simulink model "IEEE34BARRAS"  (R2018a)
settings: Solver=ode4  StartTime=0.0  StopTime=48*T  FixedStep=Ts  RelTol=1e-3  EnableMultiTasking=on
InitFcn:
  | close
  | clc
  | clear
  | n=2^8;
  | f=60;
  | T=1/f;
  | Ts=1/(f*n);
  | NT=18;
  | set_param('IEEE34BARRAS/EMISOR-RECEPTOR/TCP_IP_RX1/ESCRITURA', 'Value','[0,0,0,0,0,0,0,0,0,0,0,0,0,0,0,0,0,0,0,0,0,0,0,0,0,0,0,0,0,0,0,0,0,0,0,0,0,0,0,0,0]')
  | set_param('IEEE34BARRAS/EMISOR-RECEPTOR/TCP_IP_RX1/RETARDO', 'Value','0')
  | run script_client_1_inicio1.m
undefined symbols (not defined in the file or in its folder): D1, Delta, DiscIntNeverNeededParam, Ip1
libraries: powerlib x313, simulink x15, libreria_medidores1T x3, libreria_comunicaciones_cliente1T x2
(part 1 of 5)
settings Model: Creator=Juan Antonio Ocampo  LastModifiedBy=ana-n
settings DataIOCC: LimitDataPoints=on
settings OptimizationCC: LifeSpan=inf
settings DebuggingCC: AllowSymbolicDim=off  SFUnexpectedBacktrackingDiag=warning  SFNoUnconditionalDefaultTransitionDiag=warning  SFExecutionAtInitializationDiag=none
settings ModelReferenceCC: PropagateSignalLabelsOutOfModel=off
settings CodeAppCC: StateflowObjectComments=on
settings GRTTargetCC: TargetLangStandard=C89/C90 (ANSI)
settings ConfigComp: CovMetricSettings=dw  CovHtmlReporting=on  CovSaveCumulativeToWorkspaceVar=on  CovSaveSingleToWorkspaceVar=on  CovExternalEMLEnable=off
settings SimscapeCC: SimscapeNormalizeSystem=off

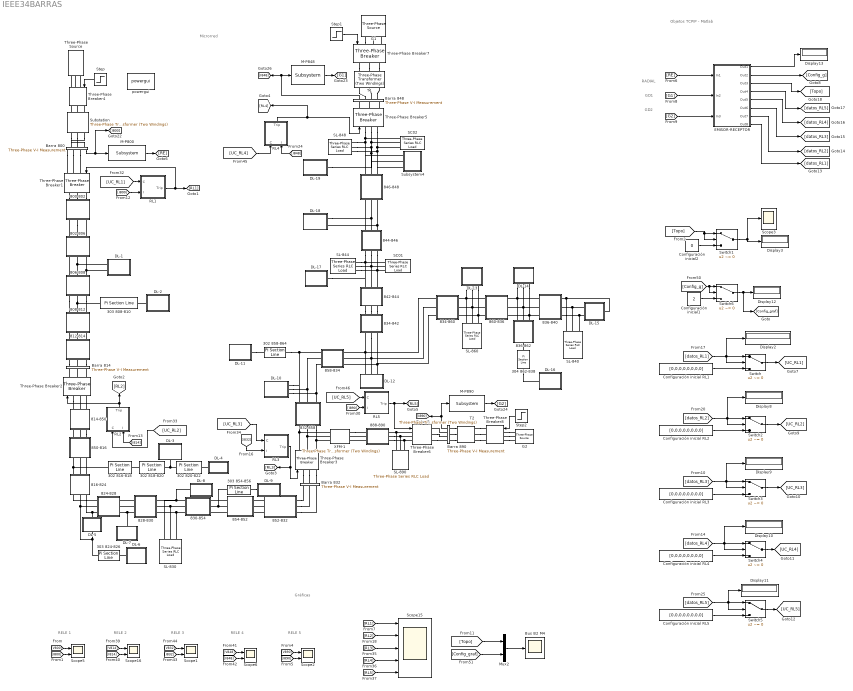
== system IEEE34BARRAS ==
  note: RADIAL
  note: RELE 1
  note: RELE 2
  note: RELE 3
  note: RELE 5
  note: RELE 4
  note: Gráficas
  note: Microrred
  note: Objetos TCPIP - Matlab
  note: GD1
  note: GD2
  " G1" : powerlib/Electrical Sources/Three-Phase Source  InternalConnection=Yg  VoltagePhases=on  Voltage=10e3/sqrt(2)  PhaseAngle=0  Voltage_phases=[480 480 480]/sqrt(3)  PhaseAngles_phases=[0 -120 +120]  Frequency=60  NonIdealSource=on  SpecifyImpedance=on  Resistance=0.8929  Inductance=16.58e-3  ShortCircuitLevel=100e6  BaseVoltage=480  XRratio=1  BusType=swing  Pref=2.324  Qref=-0.169  Prefabc=1000e6*[1 1 1]  Qrefabc=[0, 0, 0]  Qmin=0  Qmax=0
  " G2" : powerlib/Electrical Sources/Three-Phase Source  InternalConnection=Yg  VoltagePhases=on  Voltage=10e3/sqrt(2)  PhaseAngle=0  Voltage_phases=[480 480 480]  PhaseAngles_phases=[0 -120 +120]  Frequency=60  NonIdealSource=on  SpecifyImpedance=on  Resistance=0.8929  Inductance=16.58e-3  ShortCircuitLevel=100e6  BaseVoltage=480  XRratio=1  BusType=swing  Pref=2.324  Qref=-0.169  Prefabc=1000e6*[1 1 1]  Qrefabc=[0, 0, 0]  Qmin=0  Qmax=0
  302 816-818 : powerlib/Elements/Pi Section Line  LConnTagsString=__new0  RConnTagsString=__new0  Frequency=60  Resistance=1.7396  Inductance=0.0024  Capacitance=0.0070*1e-6  Length=0.5212  PiSections=1  Measurements=None
      settings: AttributesFormatString=\n  SourceProductName=Simscape Power Systems  SourceProductBaseCode=PS
  302 818-820 : powerlib/Elements/Pi Section Line  LConnTagsString=__new0  RConnTagsString=__new0  Frequency=60  Resistance=1.7396  Inductance=0.0024  Capacitance=0.0070*1e-6  Length=14.6761  PiSections=1  Measurements=None
      settings: AttributesFormatString=\n  SourceProductName=Simscape Power Systems  SourceProductBaseCode=PS
  302 820-822 : powerlib/Elements/Pi Section Line  LConnTagsString=__new0  RConnTagsString=__new0  Frequency=60  Resistance=1.7396  Inductance=0.0024  Capacitance=0.0070*1e-6  Length=4.1880  PiSections=1  Measurements=None
      settings: AttributesFormatString=\n  SourceProductName=Simscape Power Systems  SourceProductBaseCode=PS
  302 858-864 : powerlib/Elements/Pi Section Line  LConnTagsString=__new0  RConnTagsString=__new0  Frequency=60  Resistance=1.7396  Inductance=0.0024  Capacitance=0.0070*1e-6  Length=0.4938  PiSections=1  Measurements=None
      settings: AttributesFormatString=\n  SourceProductName=Simscape Power Systems  SourceProductBaseCode=PS
  303 808-810 : powerlib/Elements/Pi Section Line  LConnTagsString=__new0  RConnTagsString=__new0  Frequency=60  Resistance=1.7396  Inductance=0.0024  Capacitance=0.0070*1e-6  Length=1.769059  PiSections=1  Measurements=None
      settings: AttributesFormatString=\n  SourceProductName=Simscape Power Systems  SourceProductBaseCode=PS
  303 824-826 : powerlib/Elements/Pi Section Line  LConnTagsString=__new0  RConnTagsString=__new0  Frequency=60  Resistance=1.7396  Inductance=0.0024  Capacitance=0.0070*1e-6  Length=1.769059  PiSections=1  Measurements=None
      settings: AttributesFormatString=\n  SourceProductName=Simscape Power Systems  SourceProductBaseCode=PS
  303 854-856 : powerlib/Elements/Pi Section Line  LConnTagsString=__new0  RConnTagsString=__new0  Frequency=60  Resistance=1.7396  Inductance=0.0024  Capacitance=0.0070*1e-6  Length=7.111  PiSections=1  Measurements=None
      settings: AttributesFormatString=\n  SourceProductName=Simscape Power Systems  SourceProductBaseCode=PS
  304 862-838 : powerlib/Elements/Pi Section Line  LConnTagsString=__new0  RConnTagsString=__new0  Frequency=60  Resistance=1.1941  Inductance=0.0023  Capacitance=0.0072*1e-6  Length=1.769059  PiSections=1  Measurements=None
      settings: AttributesFormatString=\n  SourceProductName=Simscape Power Systems  SourceProductBaseCode=PS
  800-802 : Subsystem  mask{Ft=0.4886364, R=[0.8307,0.8226,0.8361], L=[0.0022,0.0022,0.0022], C=[0.0088,0.0084,0.0081].*1e-6}
      mask prompts: Ft "Distancia"; R "Resistencia p"; L "Inductancia p"; C "Capacitancia p"
      mask Display:
      | plot(0,0,100,100,[20,20,80,80,90,80,80,20,20,10],[50,40,40,50,50,50,61,61,50,50],[56,39],[55,55],[44,44],[44,55],[53,50,50],[44,48,55])
      | text(50,30,'300', 'horizontalAlignment', 'center');
      | port_label('RConn', 1, 'a')
      | port_label('RConn', 2, 'b')
      | port_label('RConn', 3, 'c')
      | port_label('LConn', 1, 'A')
      | port_label('LConn', 2, 'B')
      | port_label('LConn', 3, 'C')
  802-806 : Subsystem  mask{Ft=0.3276515, R=[0.8307,0.8226,0.8361], L=[0.0022,0.0022,0.0022], C=[0.0088,0.0084,0.0081].*1e-6}
      mask prompts: Ft "Distancia"; R "Resistencia p"; L "Inductancia p"; C "Capacitancia p"
      mask Display:
      | plot(0,0,100,100,[20,20,80,80,90,80,80,20,20,10],[50,40,40,50,50,50,61,61,50,50],[56,39],[55,55],[44,44],[44,55],[53,50,50],[44,48,55])
      | text(50,30,'300', 'horizontalAlignment', 'center');
      | port_label('RConn', 1, 'a')
      | port_label('RConn', 2, 'b')
      | port_label('RConn', 3, 'c')
      | port_label('LConn', 1, 'A')
      | port_label('LConn', 2, 'B')
      | port_label('LConn', 3, 'C')
  806-808 : Subsystem  mask{Ft=6.1041667, R=[0.8307,0.8226,0.8361], L=[0.0022,0.0022,0.0022], C=[0.0088,0.0084,0.0081].*1e-6}
      mask prompts: Ft "Distancia"; R "Resistencia p"; L "Inductancia p"; C "Capacitancia p"
      mask Display:
      | plot(0,0,100,100,[20,20,80,80,90,80,80,20,20,10],[50,40,40,50,50,50,61,61,50,50],[56,39],[55,55],[44,44],[44,55],[53,50,50],[44,48,55])
      | text(50,30,'300', 'horizontalAlignment', 'center');
      | port_label('RConn', 1, 'a')
      | port_label('RConn', 2, 'b')
      | port_label('RConn', 3, 'c')
      | port_label('LConn', 1, 'A')
      | port_label('LConn', 2, 'B')
      | port_label('LConn', 3, 'C')
  808-812 : Subsystem  mask{Ft=7.1022727, R=[0.8307,0.8226,0.8361], L=[0.0022,0.0022,0.0022], C=[0.0088,0.0084,0.0081].*1e-6}
      mask prompts: Ft "Distancia"; R "Resistencia p"; L "Inductancia p"; C "Capacitancia p"
      mask Display:
      | plot(0,0,100,100,[20,20,80,80,90,80,80,20,20,10],[50,40,40,50,50,50,61,61,50,50],[56,39],[55,55],[44,44],[44,55],[53,50,50],[44,48,55])
      | text(50,30,'300', 'horizontalAlignment', 'center');
      | port_label('RConn', 1, 'a')
      | port_label('RConn', 2, 'b')
      | port_label('RConn', 3, 'c')
      | port_label('LConn', 1, 'A')
      | port_label('LConn', 2, 'B')
      | port_label('LConn', 3, 'C')
  812-814 : Subsystem  mask{Ft=5.6306818, R=[0.8307,0.8226,0.8361], L=[0.0022,0.0022,0.0022], C=[0.0088,0.0084,0.0081].*1e-6}
      mask prompts: Ft "Distancia"; R "Resistencia p"; L "Inductancia p"; C "Capacitancia p"
      mask Display:
      | plot(0,0,100,100,[20,20,80,80,90,80,80,20,20,10],[50,40,40,50,50,50,61,61,50,50],[56,39],[55,55],[44,44],[44,55],[53,50,50],[44,48,55])
      | text(50,30,'300', 'horizontalAlignment', 'center');
      | port_label('RConn', 1, 'a')
      | port_label('RConn', 2, 'b')
      | port_label('RConn', 3, 'c')
      | port_label('LConn', 1, 'A')
      | port_label('LConn', 2, 'B')
      | port_label('LConn', 3, 'C')
  814-850 : Subsystem  mask{Ft=0.00189394, R=[1.1993,1.1904,1.1943], L=[0.0023,0.0024,0.0023], C=[0.0084,0.0081,0.0078].*1e-6}
      mask prompts: Ft "Distancia"; R "Resistencia p"; L "Inductancia p"; C "Capacitancia p"
      mask Display:
      | plot(0,0,100,100,[20,20,80,80,90,80,80,20,20,10],[50,40,40,50,50,50,61,61,50,50],[56,39],[55,55],[44,44],[44,55],[53,50,50],[44,48,55])
      | text(50,30,'301', 'horizontalAlignment', 'center');
      | port_label('RConn', 1, 'a')
      | port_label('RConn', 2, 'b')
      | port_label('RConn', 3, 'c')
      | port_label('LConn', 1, 'A')
      | port_label('LConn', 2, 'B')
      | port_label('LConn', 3, 'C')
  816-824 : Subsystem  mask{Ft=1.9337121, R=[1.1993,1.1904,1.1943], L=[0.0023,0.0024,0.0023], C=[0.0084,0.0081,0.0078].*1e-6}
      mask prompts: Ft "Distancia"; R "Resistencia p"; L "Inductancia p"; C "Capacitancia p"
      mask Display:
      | plot(0,0,100,100,[20,20,80,80,90,80,80,20,20,10],[50,40,40,50,50,50,61,61,50,50],[56,39],[55,55],[44,44],[44,55],[53,50,50],[44,48,55])
      | text(50,30,'301', 'horizontalAlignment', 'center');
      | port_label('RConn', 1, 'a')
      | port_label('RConn', 2, 'b')
      | port_label('RConn', 3, 'c')
      | port_label('LConn', 1, 'A')
      | port_label('LConn', 2, 'B')
      | port_label('LConn', 3, 'C')
  824-828 : Subsystem  mask{Ft=0.159091, R=[1.1993,1.1904,1.1943], L=[0.0023,0.0024,0.0023], C=[0.0084,0.0081,0.0078].*1e-6}
      mask prompts: Ft "Distancia"; R "Resistencia p"; L "Inductancia p"; C "Capacitancia p"
      mask Display:
      | plot(0,0,100,100,[20,20,80,80,90,80,80,20,20,10],[50,40,40,50,50,50,61,61,50,50],[56,39],[55,55],[44,44],[44,55],[53,50,50],[44,48,55])
      | text(50,30,'301', 'horizontalAlignment', 'center');
      | port_label('RConn', 1, 'a')
      | port_label('RConn', 2, 'b')
      | port_label('RConn', 3, 'c')
      | port_label('LConn', 1, 'A')
      | port_label('LConn', 2, 'B')
      | port_label('LConn', 3, 'C')
  828-830 : Subsystem  mask{Ft=3.8712121, R=[1.1081,1.1081,1.1081,1.1082], L=[0.0026858,0.0026858,0.0026858,0.0026853], C=[3.5034e-09,3.0270e-09,3.8602e-09,3.7929e-09]}
      mask prompts: Ft "Distancia"; R "Resistencia p"; L "Inductancia p"; C "Capacitancia p"
      mask Display:
      | plot(0,0,100,100,[20,20,80,80,90,80,80,20,20,10],[50,40,40,50,50,50,61,61,50,50],[56,39],[55,55],[44,44],[44,55],[53,50,50],[44,48,55])
      | text(50,30,'301', 'horizontalAlignment', 'center');
      | port_label('RConn', 1, 'a')
      | port_label('RConn', 2, 'b')
      | port_label('RConn', 3, 'c')
      | port_label('LConn', 1, 'A')
      | port_label('LConn', 2, 'B')
      | port_label('LConn', 3, 'C')
  830-854 : Subsystem  mask{Ft=0.0984848, R=[1.1993,1.1904,1.1943], L=[0.0023,0.0024,0.0023], C=[0.0084,0.0081,0.0078].*1e-6}
      mask prompts: Ft "Distancia"; R "Resistencia p"; L "Inductancia p"; C "Capacitancia p"
      mask Display:
      | plot(0,0,100,100,[20,20,80,80,90,80,80,20,20,10],[50,40,40,50,50,50,61,61,50,50],[56,39],[55,55],[44,44],[44,55],[53,50,50],[44,48,55])
      | text(50,30,'301', 'horizontalAlignment', 'center');
      | port_label('RConn', 1, 'a')
      | port_label('RConn', 2, 'b')
      | port_label('RConn', 3, 'c')
      | port_label('LConn', 1, 'A')
      | port_label('LConn', 2, 'B')
      | port_label('LConn', 3, 'C')
  832-858 : Subsystem  mask{Ft=0.9280303, R=[1.1993,1.1904,1.1943], L=[0.0023,0.0024,0.0023], C=[0.0084,0.0081,0.0078].*1e-6}
      mask prompts: Ft "Distancia"; R "Resistencia p"; L "Inductancia p"; C "Capacitancia p"
      mask Display:
      | plot(0,0,100,100,[20,20,80,80,90,80,80,20,20,10],[50,40,40,50,50,50,61,61,50,50],[56,39],[55,55],[44,44],[44,55],[53,50,50],[44,48,55])
      | text(50,30,'301', 'horizontalAlignment', 'center');
      | port_label('RConn', 1, 'a')
      | port_label('RConn', 2, 'b')
      | port_label('RConn', 3, 'c')
      | port_label('LConn', 1, 'A')
      | port_label('LConn', 2, 'B')
      | port_label('LConn', 3, 'C')
  834-842 : Subsystem  mask{Ft=0.0530303, R=[1.1993,1.1904,1.1943], L=[0.0023,0.0024,0.0023], C=[0.0084,0.0081,0.0078].*1e-6}
      mask prompts: Ft "Distancia"; R "Resistencia p"; L "Inductancia p"; C "Capacitancia p"
      mask Display:
      | plot(0,0,100,100,[20,20,80,80,90,80,80,20,20,10],[50,40,40,50,50,50,61,61,50,50],[56,39],[55,55],[44,44],[44,55],[53,50,50],[44,48,55])
      | text(50,30,'301', 'horizontalAlignment', 'center');
      | port_label('RConn', 1, 'a')
      | port_label('RConn', 2, 'b')
      | port_label('RConn', 3, 'c')
      | port_label('LConn', 1, 'A')
      | port_label('LConn', 2, 'B')
      | port_label('LConn', 3, 'C')
  834-860 : Subsystem  mask{Ft=0.3825758, R=[1.1993,1.1904,1.1943], L=[0.0023,0.0024,0.0023], C=[0.0084,0.0081,0.0078].*1e-6}
      mask prompts: Ft "Distancia"; R "Resistencia p"; L "Inductancia p"; C "Capacitancia p"
      mask Display:
      | plot(0,0,100,100,[20,20,80,80,90,80,80,20,20,10],[50,40,40,50,50,50,61,61,50,50],[56,39],[55,55],[44,44],[44,55],[53,50,50],[44,48,55])
      | text(50,30,'301', 'horizontalAlignment', 'center');
      | port_label('RConn', 1, 'a')
      | port_label('RConn', 2, 'b')
      | port_label('RConn', 3, 'c')
      | port_label('LConn', 1, 'A')
      | port_label('LConn', 2, 'B')
      | port_label('LConn', 3, 'C')
  836-840 : Subsystem  mask{Ft=0.162879, R=[1.1993,1.1904,1.1943], L=[0.0023,0.0024,0.0023], C=[0.0084,0.0081,0.0078].*1e-6}
      mask prompts: Ft "Distancia"; R "Resistencia p"; L "Inductancia p"; C "Capacitancia p"
      mask Display:
      | plot(0,0,100,100,[20,20,80,80,90,80,80,20,20,10],[50,40,40,50,50,50,61,61,50,50],[56,39],[55,55],[44,44],[44,55],[53,50,50],[44,48,55])
      | text(50,30,'301', 'horizontalAlignment', 'center');
      | port_label('RConn', 1, 'a')
      | port_label('RConn', 2, 'b')
      | port_label('RConn', 3, 'c')
      | port_label('LConn', 1, 'A')
      | port_label('LConn', 2, 'B')
      | port_label('LConn', 3, 'C')
  836-862 : Subsystem  mask{Ft=0.0530303, R=[1.1993,1.1904,1.1943], L=[0.0023,0.0024,0.0023], C=[0.0084,0.0081,0.0078].*1e-6}
      mask prompts: Ft "Distancia"; R "Resistencia p"; L "Inductancia p"; C "Capacitancia p"
      mask Display:
      | plot(0,0,100,100,[20,20,80,80,90,80,80,20,20,10],[50,40,40,50,50,50,61,61,50,50],[56,39],[55,55],[44,44],[44,55],[53,50,50],[44,48,55])
      | text(50,30,'301', 'horizontalAlignment', 'center');
      | port_label('RConn', 1, 'a')
      | port_label('RConn', 2, 'b')
      | port_label('RConn', 3, 'c')
      | port_label('LConn', 1, 'A')
      | port_label('LConn', 2, 'B')
      | port_label('LConn', 3, 'C')
  842-844 : Subsystem  mask{Ft=0.2556818, R=[1.1993,1.1904,1.1943], L=[0.0023,0.0024,0.0023], C=[0.0084,0.0081,0.0078].*1e-6}
      mask prompts: Ft "Distancia"; R "Resistencia p"; L "Inductancia p"; C "Capacitancia p"
      mask Display:
      | plot(0,0,100,100,[20,20,80,80,90,80,80,20,20,10],[50,40,40,50,50,50,61,61,50,50],[56,39],[55,55],[44,44],[44,55],[53,50,50],[44,48,55])
      | text(50,30,'301', 'horizontalAlignment', 'center');
      | port_label('RConn', 1, 'a')
      | port_label('RConn', 2, 'b')
      | port_label('RConn', 3, 'c')
      | port_label('LConn', 1, 'A')
      | port_label('LConn', 2, 'B')
      | port_label('LConn', 3, 'C')
  844-846 : Subsystem  mask{Ft=0.6893939, R=[1.1993,1.1904,1.1943], L=[0.0023,0.0024,0.0023], C=[0.0084,0.0081,0.0078].*1e-6}
      mask prompts: Ft "Distancia"; R "Resistencia p"; L "Inductancia p"; C "Capacitancia p"
      mask Display:
      | plot(0,0,100,100,[20,20,80,80,90,80,80,20,20,10],[50,40,40,50,50,50,61,61,50,50],[56,39],[55,55],[44,44],[44,55],[53,50,50],[44,48,55])
      | text(50,30,'301', 'horizontalAlignment', 'center');
      | port_label('RConn', 1, 'a')
      | port_label('RConn', 2, 'b')
      | port_label('RConn', 3, 'c')
      | port_label('LConn', 1, 'A')
      | port_label('LConn', 2, 'B')
      | port_label('LConn', 3, 'C')
  846-848 : Subsystem  mask{Ft=0.100379, R=[1.1993,1.1904,1.1943], L=[0.0023,0.0024,0.0023], C=[0.0084,0.0081,0.0078].*1e-6}
      mask prompts: Ft "Distancia"; R "Resistencia p"; L "Inductancia p"; C "Capacitancia p"
      mask Display:
      | plot(0,0,100,100,[20,20,80,80,90,80,80,20,20,10],[50,40,40,50,50,50,61,61,50,50],[56,39],[55,55],[44,44],[44,55],[53,50,50],[44,48,55])
      | text(50,30,'301', 'horizontalAlignment', 'center');
      | port_label('RConn', 1, 'a')
      | port_label('RConn', 2, 'b')
      | port_label('RConn', 3, 'c')
      | port_label('LConn', 1, 'A')
      | port_label('LConn', 2, 'B')
      | port_label('LConn', 3, 'C')
  850-816 : Subsystem  mask{Ft=0.0587121, R=[1.1993,1.1904,1.1943], L=[0.0023,0.0024,0.0023], C=[0.0084,0.0081,0.0078].*1e-6}
      mask prompts: Ft "Distancia"; R "Resistencia p"; L "Inductancia p"; C "Capacitancia p"
      mask Display:
      | plot(0,0,100,100,[20,20,80,80,90,80,80,20,20,10],[50,40,40,50,50,50,61,61,50,50],[56,39],[55,55],[44,44],[44,55],[53,50,50],[44,48,55])
      | text(50,30,'301', 'horizontalAlignment', 'center');
      | port_label('RConn', 1, 'a')
      | port_label('RConn', 2, 'b')
      | port_label('RConn', 3, 'c')
      | port_label('LConn', 1, 'A')
      | port_label('LConn', 2, 'B')
      | port_label('LConn', 3, 'C')
  852-832 : Subsystem  mask{Ft=0.00189394, R=[1.1993,1.1904,1.1943], L=[0.0023,0.0024,0.0023], C=[0.0084,0.0081,0.0078].*1e-6}
      mask prompts: Ft "Distancia"; R "Resistencia p"; L "Inductancia p"; C "Capacitancia p"
      mask Display:
      | plot(0,0,100,100,[20,20,80,80,90,80,80,20,20,10],[50,40,40,50,50,50,61,61,50,50],[56,39],[55,55],[44,44],[44,55],[53,50,50],[44,48,55])
      | text(50,30,'301', 'horizontalAlignment', 'center');
      | port_label('RConn', 1, 'a')
      | port_label('RConn', 2, 'b')
      | port_label('RConn', 3, 'c')
      | port_label('LConn', 1, 'A')
      | port_label('LConn', 2, 'B')
      | port_label('LConn', 3, 'C')
  854-852 : Subsystem  mask{Ft=6.9753788, R=[1.1993,1.1904,1.1943], L=[0.0023,0.0024,0.0023], C=[0.0084,0.0081,0.0078].*1e-6}
      mask prompts: Ft "Distancia"; R "Resistencia p"; L "Inductancia p"; C "Capacitancia p"
      mask Display:
      | plot(0,0,100,100,[20,20,80,80,90,80,80,20,20,10],[50,40,40,50,50,50,61,61,50,50],[56,39],[55,55],[44,44],[44,55],[53,50,50],[44,48,55])
      | text(50,30,'301', 'horizontalAlignment', 'center');
      | port_label('RConn', 1, 'a')
      | port_label('RConn', 2, 'b')
      | port_label('RConn', 3, 'c')
      | port_label('LConn', 1, 'A')
      | port_label('LConn', 2, 'B')
      | port_label('LConn', 3, 'C')
  858-834 : Subsystem  mask{Ft=1.104167, R=[1.1993,1.1904,1.1943], L=[0.0023,0.0024,0.0023], C=[0.0084,0.0081,0.0078].*1e-6}
      mask prompts: Ft "Distancia"; R "Resistencia p"; L "Inductancia p"; C "Capacitancia p"
      mask Display:
      | plot(0,0,100,100,[20,20,80,80,90,80,80,20,20,10],[50,40,40,50,50,50,61,61,50,50],[56,39],[55,55],[44,44],[44,55],[53,50,50],[44,48,55])
      | text(50,30,'301', 'horizontalAlignment', 'center');
      | port_label('RConn', 1, 'a')
      | port_label('RConn', 2, 'b')
      | port_label('RConn', 3, 'c')
      | port_label('LConn', 1, 'A')
      | port_label('LConn', 2, 'B')
      | port_label('LConn', 3, 'C')
  860-836 : Subsystem  mask{Ft=0.5075758, R=[1.1993,1.1904,1.1943], L=[0.0023,0.0024,0.0023], C=[0.0084,0.0081,0.0078].*1e-6}
      mask prompts: Ft "Distancia"; R "Resistencia p"; L "Inductancia p"; C "Capacitancia p"
      mask Display:
      | plot(0,0,100,100,[20,20,80,80,90,80,80,20,20,10],[50,40,40,50,50,50,61,61,50,50],[56,39],[55,55],[44,44],[44,55],[53,50,50],[44,48,55])
      | text(50,30,'301', 'horizontalAlignment', 'center');
      | port_label('RConn', 1, 'a')
      | port_label('RConn', 2, 'b')
      | port_label('RConn', 3, 'c')
      | port_label('LConn', 1, 'A')
      | port_label('LConn', 2, 'B')
      | port_label('LConn', 3, 'C')
  888-890 : Subsystem  mask{Ft=2, R=[0.8307,0.8226,0.8361], L=[0.0022,0.0022,0.0022], C=[0.0088,0.0084,0.0081].*1e-6}
      mask prompts: Ft "Distancia"; R "Resistencia p"; L "Inductancia p"; C "Capacitancia p"
      mask Display:
      | plot(0,0,100,100,[20,20,80,80,90,80,80,20,20,10],[50,40,40,50,50,50,61,61,50,50],[56,39],[55,55],[44,44],[44,55],[53,50,50],[44,48,55])
      | text(50,30,'300', 'horizontalAlignment', 'center');
      | port_label('RConn', 1, 'a')
      | port_label('RConn', 2, 'b')
      | port_label('RConn', 3, 'c')
      | port_label('LConn', 1, 'A')
      | port_label('LConn', 2, 'B')
      | port_label('LConn', 3, 'C')
  Barra 800 : powerlib/Measurements/Three-Phase V-I Measurement  VoltageMeasurement=phase-to-phase  SetLabelV=on  LabelV=V800  Vpu=off  VpuLL=off  CurrentMeasurement=yes  SetLabelI=off  LabelI=I800  Ipu=off  Pbase=100e6  Vbase=500e3  OutputType=Complex  PhasorSimulation=off  PSBequivalent=0
  Barra 814 : powerlib/Measurements/Three-Phase V-I Measurement  VoltageMeasurement=phase-to-phase  SetLabelV=on  LabelV=V814  Vpu=off  VpuLL=off  CurrentMeasurement=yes  SetLabelI=on  LabelI=I814  Ipu=off  Pbase=100e6  Vbase=500e3  OutputType=Complex  PhasorSimulation=off  PSBequivalent=0
  Barra 832 : powerlib/Measurements/Three-Phase V-I Measurement  VoltageMeasurement=phase-to-phase  SetLabelV=on  LabelV=V832  Vpu=off  VpuLL=off  CurrentMeasurement=yes  SetLabelI=on  LabelI=I832  Ipu=off  Pbase=100e6  Vbase=500e3  OutputType=Complex  PhasorSimulation=off  PSBequivalent=0
  Barra 848 : powerlib/Measurements/Three-Phase V-I Measurement  VoltageMeasurement=phase-to-phase  SetLabelV=on  LabelV=V848  Vpu=off  VpuLL=off  CurrentMeasurement=yes  SetLabelI=off  LabelI=I848  Ipu=off  Pbase=100e6  Vbase=500e3  OutputType=Complex  PhasorSimulation=off  PSBequivalent=0
  Barra 890 : powerlib/Measurements/Three-Phase V-I Measurement  VoltageMeasurement=phase-to-phase  SetLabelV=on  LabelV=V890  Vpu=off  VpuLL=off  CurrentMeasurement=yes  SetLabelI=off  LabelI=I890  Ipu=off  Pbase=100e6  Vbase=500e3  OutputType=Complex  PhasorSimulation=off  PSBequivalent=0
  Bus B2 M4 : Scope
  Configuración inicial RL{1..5} (5 alike) : Constant  Value=[0,0,0,0,0,0,0,0]
  Configuración inicial1 : Constant  Value=2
  Configuración inicial2 : Constant  Value=0
  DL-1 : Subsystem
      mask Display: disp('802-806')
  DL-10 : Subsystem
      mask Display: disp('832-858')
  DL-11 : Subsystem
      mask Display: disp('858-864')
  DL-12 : Subsystem
      mask Display: disp('858-834')
  DL-13 : Subsystem
      mask Display: disp('834-860')
  DL-14 : Subsystem
      mask Display: disp('860-836')
  DL-15 : Subsystem
      mask Display: disp('836-840')
  DL-16 : Subsystem
      mask Display: disp('862-838')
  DL-17 : Subsystem
      mask Display: disp('842-844')
  DL-18 : Subsystem
      mask Display: disp('844-846')
  DL-19 : Subsystem
      mask Display: disp('846-848')
  DL-2 : Subsystem
      mask Display: disp('808-810')
  DL-3 : Subsystem
      mask Display: disp('818-820')
  DL-4 : Subsystem
      mask Display: disp('820-822')
  DL-5 : Subsystem
      mask Display: disp('816-824')
  DL-6 : Subsystem
      mask Display: disp('824-826')
  DL-7 : Subsystem
      mask Display: disp('824-828')
  DL-8 : Subsystem
      mask Display: disp('828-830')
  DL-9 : Subsystem
      mask Display: disp('854-856')
  Display{2..3,8..13} (8 alike) : Display
  EMISOR-RECEPTOR : Subsystem
      mask Display: disp('Emisor-Receptor')
  M-P800 : libreria_medidores1T/Subsystem  SystemSampleTime=-1
  M-P848 : libreria_medidores1T/Subsystem  SystemSampleTime=-1
  M-P890 : libreria_medidores1T/Subsystem  SystemSampleTime=-1
  Mux2 : Mux  Inputs=2
  RL1 : Subsystem  mask(Proteccion de Sobrecorriente multitopologia){TCpopup1=IEC Standard Inverse, k1=0.14, alpha1=0.02, B1=0, PS1=1.20, TMS1=0.01, Tins1=0.090, Esc1=2, Vp=300, Vs=300, F=60}
      mask prompts: TCpopup1 "Caracteristica de Disparo"; k1 "k"; alpha1 "alpha"; B1 "B"; PS1 "Seteo disparo(PS)/Seteo inferior(I>)"; TMS1 "Multiplicador de Tiempo"; Tins1 "Tins"; Esc1 "Escala"; Vp "Primario CT"; Vs "Secundario CT"; F "Frecuencia"
      mask help: Proteccion de Sobrecorriente con tres topologias internas controladas por una señal de control externa.
      mask init:
      | warning('off','Simulink:Masking:Invalid_Visible_Flag')
      mask TypeOptions TCpopup1: IEC Standard Inverse | IEC Very Inverse | IEC Long Time Inverse | IEC Extremely Inverse | IEC Ultra Inverse | IEEE Moderately Inverse | IEEE Very Inverse | IEEE Extremely Inverse
      mask Callback TCpopup1:
      | switch(get_param(gcb,'TCpopup1'))
      |     case 'IEC Standard Inverse'
      |         set_param(gcb,'k1','0.14');
      |         set_param(gcb,'alpha1','0.02');
      |         set_param(gcb,'B1','0');
      |     case 'IEC Very Inverse'
      |         set_param(gcb,'k1','13.5');
      |         set_param(gcb,'alpha1','1');
      |         set_param(gcb,'B1','0');
      |     case 'IEC Long Time Inverse'
      |         set_param(gcb,'k1','120');
      |         set_param(gcb,'alpha1','1');
      |         set_param(gcb,'B1','0');
      |     case 'IEC Extremely Inverse'
      |         set_param(gcb,'k1','80');
      |         set_param(gcb,'alpha1','2');
      |         set_param(gcb,'B1','0');
      |     case 'IEC Ultra Inverse'
      |         set_param(gcb,'k1','315.2');
      |         set_param(gcb,'alpha1','2.5');
      |         set_param(gcb,'B1','0');
      |     case 'IEEE Moderately Inverse'
      |         set_param(gcb,'k1','0.0515');
      |         set_param(gcb,'alpha1','0.02');
      |         set_param(gcb,'B1','0.114');
      |     case 'IEEE Very Inverse'
      |         set_param(gcb,'k1','19.61');
      |         set_param(gcb,'alpha1','2');
      |         set_param(gcb,'B1','0.491');
      |     case 'IEEE Extremely Inverse'
      |         set_param(gcb,'k1','28.2');
      |         set_param(gcb,'alpha1','2');
      |         set_param(gcb,'B1','0.1217');
      | end
      mask DialogControl Container6 Prompt: Protecciones
      mask DialogControl Container8 Prompt: Configuración
      mask DialogControl Container9 Prompt: Proteccion 51
      mask DialogControl Container10 Prompt: Proteccion 50
      mask DialogControl Container17 Prompt: Caracteristicas Trafo Corriente
      mask Display:
      | port_label('input',1,'D');
      | port_label('input',2,'I');
      | port_label('output',1,'S');
      | text(0.62, 0.5,'50', 'horizontalAlignment', 'center');
      | text(0.62, 0.3,'51', 'horizontalAlignment', 'center');
      | plot([0.08:0.01:0.32]+0.4,[0:0.01:0.24]*0+0.40);
      | plot(0.25*sin([0:pi/20:2*pi])+0.6,0.25*cos([0:pi/20:2*pi])+0.4);
      | %Linea Salida
      | plot([0.85:0.01:1],[0:0.01:0.15]*0+0.4);
      | %Linea Corriente
      | plot([0.2:0.01:0.35],[0:0.01:0.15]*0+0.4);
      | plot([0.1:0.01:0.2],[0:0.01:0.1]*0+0.15);
      | plot([0.1:0.01:0.35]*0+0.2,[0:0.01:0.25]+0.15);
      | %Linea tension
      | plot([0.15:0.01:0.6],[0:0.01:0.45]*0+0.7);
      | plot([0:0.01:0.05]*0+0.6,[0:0.01:0.05]+0.65);
  RL2 : Subsystem  mask(Proteccion de Sobrecorriente multitopologia){TCpopup1=IEC Standard Inverse, k1=0.14, alpha1=0.02, B1=0, PS1=1.00, TMS1=0.011, Tins1=0.060, Esc1=3, Vp=187, Vs=187, F=60}
      mask prompts: TCpopup1 "Caracteristica de Disparo"; k1 "k"; alpha1 "alpha"; B1 "B"; PS1 "Seteo disparo(PS)/Seteo inferior(I>)"; TMS1 "Multiplicador de Tiempo"; Tins1 "Tins"; Esc1 "Escala"; Vp "Primario CT"; Vs "Secundario CT"; F "Frecuencia"
      mask help: Proteccion de Sobrecorriente con tres topologias internas controladas por una señal de control externa.
      mask init:
      | warning('off','Simulink:Masking:Invalid_Visible_Flag')
      mask TypeOptions TCpopup1: IEC Standard Inverse | IEC Very Inverse | IEC Long Time Inverse | IEC Extremely Inverse | IEC Ultra Inverse | IEEE Moderately Inverse | IEEE Very Inverse | IEEE Extremely Inverse
      mask Callback TCpopup1:
      | switch(get_param(gcb,'TCpopup1'))
      |     case 'IEC Standard Inverse'
      |         set_param(gcb,'k1','0.14');
      |         set_param(gcb,'alpha1','0.02');
      |         set_param(gcb,'B1','0');
      |     case 'IEC Very Inverse'
      |         set_param(gcb,'k1','13.5');
      |         set_param(gcb,'alpha1','1');
      |         set_param(gcb,'B1','0');
      |     case 'IEC Long Time Inverse'
      |         set_param(gcb,'k1','120');
      |         set_param(gcb,'alpha1','1');
      |         set_param(gcb,'B1','0');
      |     case 'IEC Extremely Inverse'
      |         set_param(gcb,'k1','80');
      |         set_param(gcb,'alpha1','2');
      |         set_param(gcb,'B1','0');
      |     case 'IEC Ultra Inverse'
      |         set_param(gcb,'k1','315.2');
      |         set_param(gcb,'alpha1','2.5');
      |         set_param(gcb,'B1','0');
      |     case 'IEEE Moderately Inverse'
      |         set_param(gcb,'k1','0.0515');
      |         set_param(gcb,'alpha1','0.02');
      |         set_param(gcb,'B1','0.114');
      |     case 'IEEE Very Inverse'
      |         set_param(gcb,'k1','19.61');
      |         set_param(gcb,'alpha1','2');
      |         set_param(gcb,'B1','0.491');
      |     case 'IEEE Extremely Inverse'
      |         set_param(gcb,'k1','28.2');
      |         set_param(gcb,'alpha1','2');
      |         set_param(gcb,'B1','0.1217');
      | end
      mask DialogControl Container6 Prompt: Protecciones
      mask DialogControl Container8 Prompt: Configuración
      mask DialogControl Container9 Prompt: Proteccion 51
      mask DialogControl Container10 Prompt: Proteccion 50
      mask DialogControl Container17 Prompt: Caracteristicas Trafo Corriente
      mask Display:
      | port_label('input',1,'D');
      | port_label('input',2,'I');
      | port_label('output',1,'S');
      | text(0.62, 0.5,'50', 'horizontalAlignment', 'center');
      | text(0.62, 0.3,'51', 'horizontalAlignment', 'center');
      | plot([0.08:0.01:0.32]+0.4,[0:0.01:0.24]*0+0.40);
      | plot(0.25*sin([0:pi/20:2*pi])+0.6,0.25*cos([0:pi/20:2*pi])+0.4);
      | %Linea Salida
      | plot([0.85:0.01:1],[0:0.01:0.15]*0+0.4);
      | %Linea Corriente
      | plot([0.2:0.01:0.35],[0:0.01:0.15]*0+0.4);
      | plot([0.1:0.01:0.2],[0:0.01:0.1]*0+0.15);
      | plot([0.1:0.01:0.35]*0+0.2,[0:0.01:0.25]+0.15);
      | %Linea tension
      | plot([0.15:0.01:0.6],[0:0.01:0.45]*0+0.7);
      | plot([0:0.01:0.05]*0+0.6,[0:0.01:0.05]+0.65);
  RL3 : Subsystem  mask(Proteccion de Sobrecorriente multitopologia){TCpopup1=IEC Standard Inverse, k1=0.14, alpha1=0.02, B1=0, PS1=0.530, TMS1=0.011, Tins1=0.015, Esc1=5, Vp=187, Vs=187, F=60}
      mask prompts: TCpopup1 "Caracteristica de Disparo"; k1 "k"; alpha1 "alpha"; B1 "B"; PS1 "Seteo disparo(PS)/Seteo inferior(I>)"; TMS1 "Multiplicador de Tiempo"; Tins1 "Tins"; Esc1 "Escala"; Vp "Primario CT"; Vs "Secundario CT"; F "Frecuencia"
      mask help: Proteccion de Sobrecorriente con tres topologias internas controladas por una señal de control externa.
      mask init:
      | warning('off','Simulink:Masking:Invalid_Visible_Flag')
      mask TypeOptions TCpopup1: IEC Standard Inverse | IEC Very Inverse | IEC Long Time Inverse | IEC Extremely Inverse | IEC Ultra Inverse | IEEE Moderately Inverse | IEEE Very Inverse | IEEE Extremely Inverse
      mask Callback TCpopup1:
      | switch(get_param(gcb,'TCpopup1'))
      |     case 'IEC Standard Inverse'
      |         set_param(gcb,'k1','0.14');
      |         set_param(gcb,'alpha1','0.02');
      |         set_param(gcb,'B1','0');
      |     case 'IEC Very Inverse'
      |         set_param(gcb,'k1','13.5');
      |         set_param(gcb,'alpha1','1');
      |         set_param(gcb,'B1','0');
      |     case 'IEC Long Time Inverse'
      |         set_param(gcb,'k1','120');
      |         set_param(gcb,'alpha1','1');
      |         set_param(gcb,'B1','0');
      |     case 'IEC Extremely Inverse'
      |         set_param(gcb,'k1','80');
      |         set_param(gcb,'alpha1','2');
      |         set_param(gcb,'B1','0');
      |     case 'IEC Ultra Inverse'
      |         set_param(gcb,'k1','315.2');
      |         set_param(gcb,'alpha1','2.5');
      |         set_param(gcb,'B1','0');
      |     case 'IEEE Moderately Inverse'
      |         set_param(gcb,'k1','0.0515');
      |         set_param(gcb,'alpha1','0.02');
      |         set_param(gcb,'B1','0.114');
      |     case 'IEEE Very Inverse'
      |         set_param(gcb,'k1','19.61');
      |         set_param(gcb,'alpha1','2');
      |         set_param(gcb,'B1','0.491');
      |     case 'IEEE Extremely Inverse'
      |         set_param(gcb,'k1','28.2');
      |         set_param(gcb,'alpha1','2');
      |         set_param(gcb,'B1','0.1217');
      | end
      mask DialogControl Container6 Prompt: Protecciones
      mask DialogControl Container8 Prompt: Configuración
      mask DialogControl Container9 Prompt: Proteccion 51
      mask DialogControl Container10 Prompt: Proteccion 50
      mask DialogControl Container17 Prompt: Caracteristicas Trafo Corriente
      mask Display:
      | port_label('input',1,'D');
      | port_label('input',2,'I');
      | port_label('output',1,'S');
      | text(0.62, 0.5,'50', 'horizontalAlignment', 'center');
      | text(0.62, 0.3,'51', 'horizontalAlignment', 'center');
      | plot([0.08:0.01:0.32]+0.4,[0:0.01:0.24]*0+0.40);
      | plot(0.25*sin([0:pi/20:2*pi])+0.6,0.25*cos([0:pi/20:2*pi])+0.4);
      | %Linea Salida
      | plot([0.85:0.01:1],[0:0.01:0.15]*0+0.4);
      | %Linea Corriente
      | plot([0.2:0.01:0.35],[0:0.01:0.15]*0+0.4);
      | plot([0.1:0.01:0.2],[0:0.01:0.1]*0+0.15);
      | plot([0.1:0.01:0.35]*0+0.2,[0:0.01:0.25]+0.15);
      | %Linea tension
      | plot([0.15:0.01:0.6],[0:0.01:0.45]*0+0.7);
      | plot([0:0.01:0.05]*0+0.6,[0:0.01:0.05]+0.65);
  RL4 : Subsystem  mask(Proteccion de Sobrecorriente multitopologia){TCpopup1=IEC Standard Inverse, k1=0.14, alpha1=0.02, B1=0, PS1=2.0, TMS1=0.200, Tins1=10.00, Esc1=100, Vp=100, Vs=100, F=60}
      mask prompts: TCpopup1 "Caracteristica de Disparo"; k1 "k"; alpha1 "alpha"; B1 "B"; PS1 "Seteo disparo(PS)/Seteo inferior(I>)"; TMS1 "Multiplicador de Tiempo"; Tins1 "Tins"; Esc1 "Escala"; Vp "Primario CT"; Vs "Secundario CT"; F "Frecuencia"
      mask help: Proteccion de Sobrecorriente con tres topologias internas controladas por una señal de control externa.
      mask init:
      | warning('off','Simulink:Masking:Invalid_Visible_Flag')
      mask TypeOptions TCpopup1: IEC Standard Inverse | IEC Very Inverse | IEC Long Time Inverse | IEC Extremely Inverse | IEC Ultra Inverse | IEEE Moderately Inverse | IEEE Very Inverse | IEEE Extremely Inverse
      mask Callback TCpopup1:
      | switch(get_param(gcb,'TCpopup1'))
      |     case 'IEC Standard Inverse'
      |         set_param(gcb,'k1','0.14');
      |         set_param(gcb,'alpha1','0.02');
      |         set_param(gcb,'B1','0');
      |     case 'IEC Very Inverse'
      |         set_param(gcb,'k1','13.5');
      |         set_param(gcb,'alpha1','1');
      |         set_param(gcb,'B1','0');
      |     case 'IEC Long Time Inverse'
      |         set_param(gcb,'k1','120');
      |         set_param(gcb,'alpha1','1');
      |         set_param(gcb,'B1','0');
      |     case 'IEC Extremely Inverse'
      |         set_param(gcb,'k1','80');
      |         set_param(gcb,'alpha1','2');
      |         set_param(gcb,'B1','0');
      |     case 'IEC Ultra Inverse'
      |         set_param(gcb,'k1','315.2');
      |         set_param(gcb,'alpha1','2.5');
      |         set_param(gcb,'B1','0');
      |     case 'IEEE Moderately Inverse'
      |         set_param(gcb,'k1','0.0515');
      |         set_param(gcb,'alpha1','0.02');
      |         set_param(gcb,'B1','0.114');
      |     case 'IEEE Very Inverse'
      |         set_param(gcb,'k1','19.61');
      |         set_param(gcb,'alpha1','2');
      |         set_param(gcb,'B1','0.491');
      |     case 'IEEE Extremely Inverse'
      |         set_param(gcb,'k1','28.2');
      |         set_param(gcb,'alpha1','2');
      |         set_param(gcb,'B1','0.1217');
      | end
      mask DialogControl Container6 Prompt: Protecciones
      mask DialogControl Container8 Prompt: Configuración
      mask DialogControl Container9 Prompt: Proteccion 51
      mask DialogControl Container10 Prompt: Proteccion 50
      mask DialogControl Container17 Prompt: Caracteristicas Trafo Corriente
      mask Display:
      | port_label('input',1,'D');
      | port_label('input',2,'I');
      | port_label('output',1,'S');
      | text(0.62, 0.5,'50', 'horizontalAlignment', 'center');
      | text(0.62, 0.3,'51', 'horizontalAlignment', 'center');
      | plot([0.08:0.01:0.32]+0.4,[0:0.01:0.24]*0+0.40);
      | plot(0.25*sin([0:pi/20:2*pi])+0.6,0.25*cos([0:pi/20:2*pi])+0.4);
      | %Linea Salida
      | plot([0.85:0.01:1],[0:0.01:0.15]*0+0.4);
      | %Linea Corriente
      | plot([0.2:0.01:0.35],[0:0.01:0.15]*0+0.4);
      | plot([0.1:0.01:0.2],[0:0.01:0.1]*0+0.15);
      | plot([0.1:0.01:0.35]*0+0.2,[0:0.01:0.25]+0.15);
      | %Linea tension
      | plot([0.15:0.01:0.6],[0:0.01:0.45]*0+0.7);
      | plot([0:0.01:0.05]*0+0.6,[0:0.01:0.05]+0.65);
  RL5 : Subsystem  mask(Proteccion de Sobrecorriente multitopologia){TCpopup1=IEC Standard Inverse, k1=0.14, alpha1=0.02, B1=0, PS1=2.0, TMS1=0.200, Tins1=10.0, Esc1=100, Vp=10, Vs=10, F=60}
      mask prompts: TCpopup1 "Caracteristica de Disparo"; k1 "k"; alpha1 "alpha"; B1 "B"; PS1 "Seteo disparo(PS)/Seteo inferior(I>)"; TMS1 "Multiplicador de Tiempo"; Tins1 "Tins"; Esc1 "Escala"; Vp "Primario CT"; Vs "Secundario CT"; F "Frecuencia"
      mask help: Proteccion de Sobrecorriente con tres topologias internas controladas por una señal de control externa.
      mask init:
      | warning('off','Simulink:Masking:Invalid_Visible_Flag')
      mask TypeOptions TCpopup1: IEC Standard Inverse | IEC Very Inverse | IEC Long Time Inverse | IEC Extremely Inverse | IEC Ultra Inverse | IEEE Moderately Inverse | IEEE Very Inverse | IEEE Extremely Inverse
      mask Callback TCpopup1:
      | switch(get_param(gcb,'TCpopup1'))
      |     case 'IEC Standard Inverse'
      |         set_param(gcb,'k1','0.14');
      |         set_param(gcb,'alpha1','0.02');
      |         set_param(gcb,'B1','0');
      |     case 'IEC Very Inverse'
      |         set_param(gcb,'k1','13.5');
      |         set_param(gcb,'alpha1','1');
      |         set_param(gcb,'B1','0');
      |     case 'IEC Long Time Inverse'
      |         set_param(gcb,'k1','120');
      |         set_param(gcb,'alpha1','1');
      |         set_param(gcb,'B1','0');
      |     case 'IEC Extremely Inverse'
      |         set_param(gcb,'k1','80');
      |         set_param(gcb,'alpha1','2');
      |         set_param(gcb,'B1','0');
      |     case 'IEC Ultra Inverse'
      |         set_param(gcb,'k1','315.2');
      |         set_param(gcb,'alpha1','2.5');
      |         set_param(gcb,'B1','0');
      |     case 'IEEE Moderately Inverse'
      |         set_param(gcb,'k1','0.0515');
      |         set_param(gcb,'alpha1','0.02');
      |         set_param(gcb,'B1','0.114');
      |     case 'IEEE Very Inverse'
      |         set_param(gcb,'k1','19.61');
      |         set_param(gcb,'alpha1','2');
      |         set_param(gcb,'B1','0.491');
      |     case 'IEEE Extremely Inverse'
      |         set_param(gcb,'k1','28.2');
      |         set_param(gcb,'alpha1','2');
      |         set_param(gcb,'B1','0.1217');
      | end
      mask DialogControl Container6 Prompt: Protecciones
      mask DialogControl Container8 Prompt: Configuración
      mask DialogControl Container9 Prompt: Proteccion 51
      mask DialogControl Container10 Prompt: Proteccion 50
      mask DialogControl Container17 Prompt: Caracteristicas Trafo Corriente
      mask Display:
      | port_label('input',1,'D');
      | port_label('input',2,'I');
      | port_label('output',1,'S');
      | text(0.62, 0.5,'50', 'horizontalAlignment', 'center');
      | text(0.62, 0.3,'51', 'horizontalAlignment', 'center');
      | plot([0.08:0.01:0.32]+0.4,[0:0.01:0.24]*0+0.40);
      | plot(0.25*sin([0:pi/20:2*pi])+0.6,0.25*cos([0:pi/20:2*pi])+0.4);
      | %Linea Salida
      | plot([0.85:0.01:1],[0:0.01:0.15]*0+0.4);
      | %Linea Corriente
      | plot([0.2:0.01:0.35],[0:0.01:0.15]*0+0.4);
      | plot([0.1:0.01:0.2],[0:0.01:0.1]*0+0.15);
      | plot([0.1:0.01:0.35]*0+0.2,[0:0.01:0.25]+0.15);
      | %Linea tension
      | plot([0.15:0.01:0.6],[0:0.01:0.45]*0+0.7);
      | plot([0:0.01:0.05]*0+0.6,[0:0.01:0.05]+0.65);
  SC01 : powerlib/Elements/Three-Phase Series RLC Load  LConnTagsString=A|B|C  Configuration=Delta  NominalVoltage=24.9e3  Vabc=[14.376e3,14.376e3,14.376e3]  Vabcp=[1e3 1e3 1e3]  NominalFrequency=60  UnbalancedPower=off  ActivePower=0  InductivePower=0  CapacitivePower=100  Pabc=[0 25e3 20e3]  QLabc=[0 12e3 11e3]  QCabc=[0 0 0]  Pabcp=[10e3 9e3 11e3]  QLabcp=[100 90 110]  QCabcp=[100 90 110]  Measurements=None  LoadType=constant PQ
  SC02 : powerlib/Elements/Three-Phase Series RLC Load  LConnTagsString=A|B|C  Configuration=Delta  NominalVoltage=24.9e3  Vabc=[14.376e3,14.376e3,14.376e3]  Vabcp=[1e3 1e3 1e3]  NominalFrequency=60  UnbalancedPower=off  ActivePower=0  InductivePower=0  CapacitivePower=150  Pabc=[0 25e3 20e3]  QLabc=[0 12e3 11e3]  QCabc=[0 0 0]  Pabcp=[10e3 9e3 11e3]  QLabcp=[100 90 110]  QCabcp=[100 90 110]  Measurements=None  LoadType=constant PQ
  SL-830 : powerlib/Elements/Three-Phase Series RLC Load  LConnTagsString=A|B|C  Configuration=Delta  NominalVoltage=24.9e3  Vabc=[14.376e3,14.376e3,14.376e3]  Vabcp=[24.9e3 24.9e3 24.9e3]  NominalFrequency=60  UnbalancedPower=on  ActivePower=150e3  InductivePower=75e3  CapacitivePower=0  Pabc=[20e3 20e3 20e3]  QLabc=[16e3 16e3 16e3]  QCabc=[0 0 0]  Pabcp=[10e3 10e3 25e3]  QLabcp=[5e3 5e3 10e3]  QCabcp=[0 0 0]  Measurements=None  LoadType=constant Z
  SL-840 : powerlib/Elements/Three-Phase Series RLC Load  LConnTagsString=A|B|C  Configuration=Y (grounded)  NominalVoltage=1000  Vabc=[14.376e3,14.376e3,14.376e3]  Vabcp=[1e3 1e3 1e3]  NominalFrequency=60  UnbalancedPower=on  ActivePower=10e3  InductivePower=100  CapacitivePower=0  Pabc=[9e3 9e3 9e3]  QLabc=[7e3 7e3 7e3]  QCabc=[0 0 0]  Pabcp=[10e3 9e3 11e3]  QLabcp=[100 90 110]  QCabcp=[100 90 110]  Measurements=None  LoadType=constant I
  SL-844 : powerlib/Elements/Three-Phase Series RLC Load  LConnTagsString=A|B|C  Configuration=Y (grounded)  NominalVoltage=1000  Vabc=[14.376e3,14.376e3,14.376e3]  Vabcp=[1e3 1e3 1e3]  NominalFrequency=60  UnbalancedPower=on  ActivePower=10e3  InductivePower=100  CapacitivePower=0  Pabc=[135e3 135e3 135e3]  QLabc=[105e3 105e3 105e3]  QCabc=[0 0 0]  Pabcp=[10e3 9e3 11e3]  QLabcp=[100 90 110]  QCabcp=[100 90 110]  Measurements=None  LoadType=constant Z
  SL-848 : powerlib/Elements/Three-Phase Series RLC Load  LConnTagsString=A|B|C  Configuration=Delta  NominalVoltage=1000  Vabc=[14.376e3,14.376e3,14.376e3]  Vabcp=[24.9e3 24.9e3 24.9e3]  NominalFrequency=60  UnbalancedPower=on  ActivePower=10e3  InductivePower=100  CapacitivePower=0  Pabc=[20e3 20e3 20e3]  QLabc=[16e3 16e3 16e3]  QCabc=[0 0 0]  Pabcp=[20e3 20e3 20e3]  QLabcp=[16e3 16e3 16e3]  QCabcp=[0 0 0]  Measurements=None  LoadType=constant PQ
  SL-860 : powerlib/Elements/Three-Phase Series RLC Load  LConnTagsString=A|B|C  Configuration=Y (grounded)  NominalVoltage=1000  Vabc=[14.376e3,14.376e3,14.376e3]  Vabcp=[1e3 1e3 1e3]  NominalFrequency=60  UnbalancedPower=on  ActivePower=10e3  InductivePower=100  CapacitivePower=0  Pabc=[20e3 20e3 20e3]  QLabc=[16e3 16e3 16e3]  QCabc=[0 0 0]  Pabcp=[10e3 9e3 11e3]  QLabcp=[100 90 110]  QCabcp=[100 90 110]  Measurements=None  LoadType=constant PQ
  SL-890 : powerlib/Elements/Three-Phase Series RLC Load  LConnTagsString=A|B|C  Configuration=Delta  NominalVoltage=1000  Vabc=[14.376e3,14.376e3,14.376e3]  Vabcp=[4.16e3 4.16e3 4.16e3]  NominalFrequency=60  UnbalancedPower=off  ActivePower=150e3  InductivePower=75e3  CapacitivePower=0  Pabc=[20e3 20e3 20e3]  QLabc=[16e3 16e3 16e3]  QCabc=[0 0 0]  Pabcp=[20e3 20e3 20e3]  QLabcp=[16e3 16e3 16e3]  QCabcp=[0 0 0]  Measurements=None  LoadType=constant I
  Scope{1..2,5..6,16} (5 alike) : Scope  NumInputPorts=2
  Scope15 : Scope  NumInputPorts=5
  Scope3 : Scope
  Step : Step  Time=10  Before=1  After=0  SampleTime=0
  Step1 : Step  Time=0.2  Before=1  After=0  SampleTime=0
  Step2 : Step  Time=0.2  Before=1  After=0  SampleTime=0
  Substation : powerlib/Elements/Three-Phase Transformer (Two Windings)  Winding1Connection=Delta (D1)  Winding2Connection=Yg  CoreType=Three single-phase transformers  SetSaturation=off  Hysteresis=off  DataFile='hysteresis'  SetInitialFlux=off  Measurements=None  UNITS=SI  NominalPower=[2500e3 , 60 ]  Winding1=[69e3 0.000001 0.000001]  Winding2=[24.9e3 2.48 19.8403/377]  Rm=1.0805e+06  Lm=2866  L0=0.5  Saturation=[0 0;0.66653 1910.3;277.72 2419.7]  InitialFluxes=[1273.5 -1273.5 1114.3]  MoreParameters=off  BreakLoop=off  DataType=on  TransfoNumber=1
  Subsystem4 : Subsystem
      mask Display: disp('F6')
  Switch{,1..6} (7 alike) : Switch  Criteria=u2 ~= 0
  T1 : powerlib/Elements/Three-Phase Transformer (Two Windings)  Winding1Connection=Yg  Winding2Connection=Yg  CoreType=Three single-phase transformers  SetSaturation=off  Hysteresis=off  DataFile='hysteresis'  SetInitialFlux=off  Measurements=None  UNITS=SI  NominalPower=[ 750e3 , 60 ]  Winding1=[24.9e3 0.000001 0.000001]  Winding2=[0.48e3 0.0031 0.0154/377]  Rm=1.0805e+06  Lm=2866  L0=0.5  Saturation=[0 0;0.66653 1910.3;277.72 2419.7]  InitialFluxes=[1273.5 -1273.5 1114.3]  MoreParameters=off  BreakLoop=off  DataType=on  TransfoNumber=1
  T2 : powerlib/Elements/Three-Phase Transformer (Two Windings)  Winding1Connection=Yg  Winding2Connection=Yg  CoreType=Three single-phase transformers  SetSaturation=off  Hysteresis=off  DataFile='hysteresis'  SetInitialFlux=off  Measurements=None  UNITS=SI  NominalPower=[ 750e3 , 60 ]  Winding1=[4.16e3 0.000001 0.000001]  Winding2=[0.48e3 0.0031 0.0154]  Rm=1.0805e+06  Lm=2866  L0=0.5  Saturation=[0 0;0.66653 1910.3;277.72 2419.7]  InitialFluxes=[1273.5 -1273.5 1114.3]  MoreParameters=off  BreakLoop=off  DataType=on  TransfoNumber=1
  Three-Phase Breaker{1..3,5..8} (7 alike) : powerlib/Elements/Three-Phase Breaker  InitialState=closed  SwitchA=on  SwitchB=on  SwitchC=on  SwitchTimes="[1/60  5/60]"  External=on  BreakerResistance=0.01  SnubberResistance=1e6  SnubberCapacitance=inf  Measurements=None
  Three-Phase Breaker4 : powerlib/Elements/Three-Phase Breaker  InitialState=open  SwitchA=on  SwitchB=on  SwitchC=on  SwitchTimes="[1/60  5/60]"  External=on  BreakerResistance=0.01  SnubberResistance=1e6  SnubberCapacitance=inf  Measurements=None
  Three-Phase Source : powerlib/Electrical Sources/Three-Phase Source  InternalConnection=Yg  VoltagePhases=off  Voltage=69e3  PhaseAngle=0  Voltage_phases=[25e3 25e3 25e3]/sqrt(3)  PhaseAngles_phases=[0 -120 +120]  Frequency=60  NonIdealSource=on  SpecifyImpedance=off  Resistance=0.8929  Inductance=16.58e-3  ShortCircuitLevel=100e6  BaseVoltage=25e3  XRratio=7  BusType=swing  Pref=10e3  Qref=0  Prefabc=[10e3, 10e3, 10e3]  Qrefabc=[0, 0, 0]  Qmin=-inf  Qmax=inf
  XFM-1 : powerlib/Elements/Three-Phase Transformer (Two Windings)  Winding1Connection=Yg  Winding2Connection=Yg  CoreType=Three single-phase transformers  SetSaturation=off  Hysteresis=off  DataFile='hysteresis'  SetInitialFlux=off  Measurements=None  UNITS=SI  NominalPower=[500e3 , 60 ]  Winding1=[24.9e3 23.5600 50.5920/377]  Winding2=[4.16e3 0.000001 0.000001]  Rm=1.0805e+06  Lm=2866  L0=0.5  Saturation=[0 0;0.66653 1910.3;277.72 2419.7]  InitialFluxes=[1273.5 -1273.5 1114.3]  MoreParameters=off  BreakLoop=off  DataType=on  TransfoNumber=1
  powergui : powerlib/powergui  Priority=1  SimulationMode=Discrete  SampleTime=Ts  frequency=60  Iterations=50  frequencyindice=0  Pbase=100e6  ErrMax=1e-4  UnitsV=kV  UnitsW=MW  buscounter=0  FunctionMessages=off  echomessages=off  EnableUseOfTLC=off  CurrentSourceSwitches=off  DisableSnubberDevices=off  DisableRonSwitches=off  DisableVfSwitches=off  DisplayEquations=off  SolverType=Tustin/Backward Euler (TBE)  Interpol=off  ExternalGateDelay=off  methode=off  Ts=10  x0status=blocks  SPID=off  SwTol=0  HookPort=off  RestoreLinks=warning  ResistiveCurrentMeasurement=off  Frange=[0:2:500]  Ylog=off  Xlog=on  ShowGrid=off  save=off  variable=ZData  structure=0  ZoomFFT=off  StartTime=0.0  cycles=1  DisplayStyle=1  fundamental=60  FreqAxis=off  MaxFrequency=1000  frequencyindicesteady=1  RmsSteady=1  display=off
  wires:
  [V800] -> Scope5/1
  [I800] -> Scope5/2
  [I814] -> RL2/2(I)
  RL1/1(Trip) -> [RL1], Three-Phase Breaker1/1
  RL2/1(Trip) -> [RL2], Three-Phase Breaker2/1
  [I800] -> RL1/2(I)
  RL3/1(Trip) -> Three-Phase Breaker3/1, [RL3]
  [I848] -> RL4/2(I)
  RL4/1(Trip) -> Three-Phase Breaker5/1, [RL4]
  RL5/1(Trip) -> [RL5], Three-Phase Breaker6/1
  [UC_RL4] -> RL4/1(C)
  [UC_RL3] -> RL3/1(C)
  [UC_RL5] -> RL5/1(C)
  [I890] -> RL5/2(I)
  [I832] -> RL3/2(I)
  [RL5] -> Scope15/5
  [RL2] -> Scope15/2
  [RL1] -> Scope15/1
  [RL3] -> Scope15/3
  [RL4] -> Scope15/4
  [V814] -> Scope16/1
  [I814] -> Scope16/2
  [V890] -> Scope2/1
  [I890] -> Scope2/2
  [I832] -> Scope1/2
  [V832] -> Scope1/1
  [I848] -> Scope6/2
  [V848] -> Scope6/1
  Switch/1 -> [UC_RL1]
  Configuración inicial RL1/1 -> Switch/3
  Step/1 -> Three-Phase Breaker4/1
  Step1/1 -> Three-Phase Breaker7/1
  Step2/1 -> Three-Phase Breaker8/1
  Configuración inicial2/1 -> Switch1/3
  Configuración inicial RL2/1 -> Switch2/3
  Switch2/1 -> [UC_RL2]
  Switch3/1 -> [UC_RL3]
  Configuración inicial RL3/1 -> Switch3/3
  Configuración inicial RL5/1 -> Switch5/3
  Switch5/1 -> [UC_RL5]
  Switch4/1 -> [UC_RL4]
  Configuración inicial RL4/1 -> Switch4/3
  [datos_RL1] -> Switch/2, Display2/1, Switch/1
  [datos_RL2] -> Switch2/2, Display8/1, Switch2/1
  [datos_RL4] -> Switch4/2, Display10/1, Switch4/1
  [datos_RL5] -> Switch5/2, Display11/1, Switch5/1
  [datos_RL3] -> Switch3/2, Display9/1, Switch3/1
  [UC_RL2] -> RL2/1(C)
  [UC_RL1] -> RL1/1(C)
  [Topo] -> Mux2/1
  [Config_graf] -> Mux2/2
  Mux2/1 -> Bus B2 M4/1
  Switch1/1 -> Display3/1, Scope3/1
  [Config_g] -> Switch6/2, Switch6/1
  Configuración inicial1/1 -> Switch6/3
  Switch6/1 -> [Config_graf], Display12/1
  M-P800/1 -> [RE]
  Barra 800/1 -> [I800], M-P800/1
  M-P890/1 -> [G2]
  Barra 890/1 -> M-P890/1, [I890]
  Barra 848/1 -> M-P848/1, [I848]
  M-P848/1 -> [G1]
  EMISOR-RECEPTOR/3(Out3) -> [Topo]
  [RE] -> EMISOR-RECEPTOR/1(In1)
  [G1] -> EMISOR-RECEPTOR/2(In2)
  [G2] -> EMISOR-RECEPTOR/3(In3)
  EMISOR-RECEPTOR/1(Out1) -> Display13/1
  EMISOR-RECEPTOR/2(Out2) -> [Config_g]
  EMISOR-RECEPTOR/4(Out4) -> [datos_RL5]
  EMISOR-RECEPTOR/5(Out5) -> [datos_RL4]
  EMISOR-RECEPTOR/6(Out6) -> [datos_RL3]
  EMISOR-RECEPTOR/7(Out7) -> [datos_RL2]
  EMISOR-RECEPTOR/8(Out8) -> [datos_RL1]
  [Topo] -> Switch1/2, Switch1/1
  connections:
  806-808/LConn1 -- 802-806/RConn1
  806-808/LConn2 -- DL-1/RConn1 -- 802-806/RConn2
  806-808/LConn3 -- 802-806/RConn3 -- DL-1/RConn2
  806-808/RConn1 -- 808-812/LConn1
  806-808/RConn2 -- 808-812/LConn2 -- 303 808-810/RConn1
  806-808/RConn3 -- 808-812/LConn3
  812-814/LConn1 -- 808-812/RConn1
  812-814/LConn2 -- 808-812/RConn2
  812-814/LConn3 -- 808-812/RConn3
  850-816/LConn2 -- 814-850/RConn2
  816-824/LConn1 -- 850-816/RConn1 -- 302 816-818/LConn1
  816-824/LConn2 -- 850-816/RConn2
  816-824/LConn3 -- 850-816/RConn3
  824-828/LConn2 -- 303 824-826/LConn1 -- DL-5/LConn1 -- 816-824/RConn2
  828-830/LConn2 -- 824-828/RConn2
  830-854/LConn1 -- 828-830/RConn1 -- SL-830/LConn1 -- DL-8/LConn1
  830-854/LConn2 -- 828-830/RConn2 -- SL-830/LConn2
  830-854/LConn3 -- SL-830/LConn3 -- 828-830/RConn3
  303 854-856/LConn1 -- 854-852/LConn2 -- 830-854/RConn2
  832-858/LConn1 -- XFM-1/LConn1 -- Three-Phase Breaker3/RConn1
  832-858/LConn2 -- XFM-1/LConn2 -- Three-Phase Breaker3/RConn2
  858-834/LConn1 -- 832-858/RConn1 -- DL-10/LConn1 -- 302 858-864/LConn1
  842-844/LConn1 -- 834-842/RConn1
  842-844/LConn2 -- 834-842/RConn2
  842-844/LConn3 -- 834-842/RConn3
  844-846/LConn2 -- SC01/LConn2 -- SL-844/LConn2 -- 842-844/RConn2
  844-846/LConn3 -- SC01/LConn3 -- SL-844/LConn3 -- 842-844/RConn3
  860-836/LConn2 -- DL-13/LConn2 -- SL-860/LConn2 -- 834-860/RConn2
  860-836/LConn3 -- DL-13/LConn3 -- SL-860/LConn3 -- 834-860/RConn3
  836-840/LConn1 -- DL-14/LConn1 -- 836-862/LConn1 -- 860-836/RConn1
  836-840/LConn2 -- DL-14/LConn2 -- 836-862/LConn2 -- 860-836/RConn2
  836-840/LConn3 -- DL-14/LConn3 -- 836-862/LConn3 -- 860-836/RConn3
  888-890/LConn3 -- XFM-1/RConn3
  836-840/RConn1 -- SL-840/LConn1 -- DL-15/RConn1
  SL-840/LConn2 -- DL-15/LConn1 -- 836-840/RConn2
  SL-840/LConn3 -- 836-840/RConn3 -- DL-15/LConn2
  SL-848/LConn1 -- Three-Phase Breaker5/LConn1 -- SC02/LConn1 -- Subsystem4/LConn1 -- 846-848/RConn1
  SL-848/LConn3 -- Three-Phase Breaker5/LConn3 -- SC02/LConn3 -- Subsystem4/LConn3 -- 846-848/RConn3
  888-890/RConn2 -- Three-Phase Breaker6/LConn2 -- SL-890/LConn2
  888-890/RConn3 -- Three-Phase Breaker6/LConn3 -- SL-890/LConn3
  DL-10/LConn2 -- 858-834/LConn2 -- 832-858/RConn2
  DL-10/LConn3 -- 858-834/LConn3 -- 832-858/RConn3
  Three-Phase Breaker1/RConn2 -- 800-802/LConn2
  Three-Phase Breaker1/RConn1 -- 800-802/LConn3
  832-858/LConn3 -- XFM-1/LConn3 -- Three-Phase Breaker3/RConn3
  802-806/LConn1 -- 800-802/RConn1
  800-802/RConn2 -- 802-806/LConn2
  802-806/LConn3 -- 800-802/RConn3
  812-814/RConn1 -- Barra 814/LConn3
  Barra 814/LConn2 -- 812-814/RConn2
  812-814/RConn3 -- Barra 814/LConn1
  302 818-820/LConn1 -- 302 816-818/RConn1
  852-832/RConn3 -- Barra 832/RConn1
  852-832/RConn2 -- Barra 832/RConn2
  852-832/RConn1 -- Barra 832/RConn3
  DL-12/LConn2 -- 834-842/LConn2 -- 858-834/RConn2 -- 834-860/LConn2
  888-890/LConn2 -- XFM-1/RConn2
  304 862-838/LConn1 -- 836-862/RConn2
  Substation/RConn1 -- Barra 800/LConn3
  Substation/RConn3 -- Barra 800/LConn1
  Substation/RConn2 -- Barra 800/LConn2
  844-846/RConn1 -- 846-848/LConn1
  DL-18/RConn1 -- 846-848/LConn2 -- 844-846/RConn2
  844-846/RConn3 -- 846-848/LConn3 -- DL-18/RConn2
  Barra 800/RConn1 -- Three-Phase Breaker1/LConn1
  Barra 800/RConn2 -- Three-Phase Breaker1/LConn2
  Barra 800/RConn3 -- Three-Phase Breaker1/LConn3
  814-850/RConn3 -- 850-816/LConn3
  Three-Phase Breaker1/RConn3 -- 800-802/LConn1
  Three-Phase Breaker2/LConn1 -- 814-850/LConn1
  814-850/LConn2 -- Three-Phase Breaker2/LConn2
  814-850/LConn3 -- Three-Phase Breaker2/LConn3
  Three-Phase Breaker2/RConn1 -- Barra 814/RConn3
  Three-Phase Breaker2/RConn2 -- Barra 814/RConn2
  Three-Phase Breaker2/RConn3 -- Barra 814/RConn1
  SL-890/LConn1 -- 888-890/RConn1 -- Three-Phase Breaker6/LConn1
  816-824/RConn3 -- DL-5/RConn1 -- 824-828/LConn3
  816-824/RConn1 -- 824-828/LConn1
  828-830/LConn1 -- 824-828/RConn1
  824-828/RConn3 -- 828-830/LConn3 -- DL-7/LConn1
  DL-12/LConn3 -- 834-860/LConn3 -- 834-842/LConn3 -- 858-834/RConn3
  DL-12/LConn1 -- 834-842/LConn1 -- 858-834/RConn1 -- 834-860/LConn1
  XFM-1/RConn1 -- 888-890/LConn1
  Three-Phase Breaker3/LConn1 -- Barra 832/LConn3
  Three-Phase Breaker3/LConn2 -- Barra 832/LConn2
  Three-Phase Breaker3/LConn3 -- Barra 832/LConn1
  T1/LConn1 -- Barra 848/RConn1
  Barra 848/LConn2 -- Three-Phase Breaker5/RConn2
  Three-Phase Breaker5/RConn1 -- Barra 848/LConn1
  Three-Phase Breaker5/RConn3 -- Barra 848/LConn3
  Barra 848/RConn2 -- T1/LConn2
  Barra 848/RConn3 -- T1/LConn3
  DL-2/LConn1 -- 303 808-810/LConn1
  DL-4/LConn1 -- 302 820-822/RConn1
  302 820-822/LConn1 -- DL-3/LConn1 -- 302 818-820/RConn1
  850-816/LConn1 -- 814-850/RConn1
  DL-6/LConn1 -- 303 824-826/RConn1
  303 854-856/RConn1 -- DL-9/LConn1
  304 862-838/RConn1 -- DL-16/LConn1
  SL-860/LConn1 -- 860-836/LConn1 -- DL-13/LConn1 -- 834-860/RConn1
  844-846/LConn1 -- SL-844/LConn1 -- DL-17/LConn1 -- 842-844/RConn1 -- SC01/LConn1
  Three-Phase Breaker5/LConn2 -- Subsystem4/LConn2 -- DL-19/LConn1 -- 846-848/RConn2 -- SL-848/LConn2 -- SC02/LConn2
  854-852/LConn3 -- 830-854/RConn3
  854-852/LConn1 -- 830-854/RConn1
  852-832/LConn1 -- 854-852/RConn1
  852-832/LConn2 -- 854-852/RConn2
  852-832/LConn3 -- 854-852/RConn3
  Barra 890/RConn1 -- Three-Phase Breaker6/RConn1
  Three-Phase Breaker6/RConn2 -- Barra 890/RConn2
  Three-Phase Breaker6/RConn3 -- Barra 890/RConn3
  Barra 890/LConn1 -- T2/LConn1
  Barra 890/LConn2 -- T2/LConn2
  Barra 890/LConn3 -- T2/LConn3
  DL-11/LConn1 -- 302 858-864/RConn1
  Three-Phase Breaker4/LConn3 -- Three-Phase Source/RConn3
  Three-Phase Breaker4/RConn3 -- Substation/LConn3
  Three-Phase Breaker4/RConn2 -- Substation/LConn2
  Three-Phase Breaker4/RConn1 -- Substation/LConn1
  Three-Phase Breaker4/LConn1 -- Three-Phase Source/RConn1
  Three-Phase Breaker4/LConn2 -- Three-Phase Source/RConn2
  Three-Phase Breaker7/LConn2 -- " G1"/RConn2
  Three-Phase Breaker7/LConn3 -- " G1"/RConn3
  Three-Phase Breaker7/RConn2 -- T1/RConn2
  Three-Phase Breaker7/RConn1 -- T1/RConn1
  Three-Phase Breaker7/RConn3 -- T1/RConn3
  " G1"/RConn1 -- Three-Phase Breaker7/LConn1
  Three-Phase Breaker8/LConn3 -- " G2"/RConn3
  Three-Phase Breaker8/LConn1 -- " G2"/RConn1
  Three-Phase Breaker8/LConn2 -- " G2"/RConn2
  T2/RConn1 -- Three-Phase Breaker8/RConn1
  T2/RConn2 -- Three-Phase Breaker8/RConn2
  T2/RConn3 -- Three-Phase Breaker8/RConn3
